simulink model "dspwwv_receiver"  (Simulink 8.3)
settings: Solver=FixedStepDiscrete  StartTime=0.0  StopTime=0  RelTol=1e-3
model workspace (MATLAB code in the model file):
  | MISS = boolean(zeros(1,100)');
  | ZERO =  boolean([ones(1,17) zeros(1,83)]');
  | ONE =  boolean([ones(1,47) zeros(1,53)]');
  | MARKER =  boolean([ones(1,77) zeros(1,23)]');
undefined symbols (not defined in the file or in its folder): magnitude
libraries: dspsigops x9, dspstat3 x2, dspmlti4 x2, dspbuff3 x2, simulink x2, dspsrcs4 x1, dspswit3 x1
settings Model: Creator=The MathWorks Inc.
settings SolverCC: InsertRTBMode=Auto
settings DataIOCC: SaveFormat=Structure
settings OptimizationCC: InlineParams=on  ExpressionDepthLimit=2147483647  InitFltsAndDblsToZero=on  EfficientMapNaN2IntZero=off
settings DebuggingCC: FcnCallInpInsideContextMsg=UseLocalSettings  StrictBusMsg=Warning
settings HardwareCC: ProdIntDivRoundTo=Zero  ProdHWDeviceType=Generic->Unspecified (assume 32-bit Generic)  TargetHWDeviceType=32-bit Generic
settings ModelReferenceCC: ModelReferenceNumInstancesAllowed=Single
settings SFSimCC: SFSimEcho=off  SimParseCustomCode=off

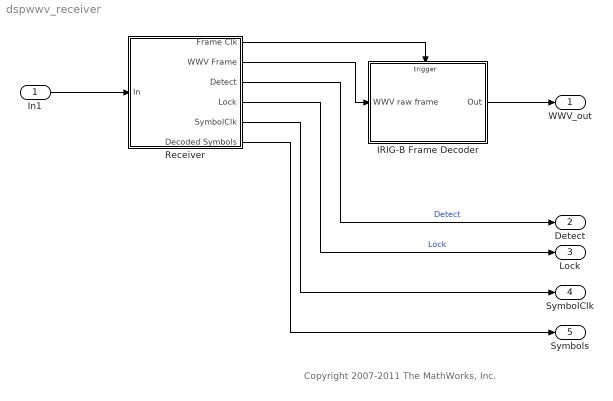
== system dspwwv_receiver ==
  note: Copyright 2007-2011 The MathWorks, Inc.
  In1 : Inport  OutDataTypeStr=single  PortDimensions=[80 1]
  IRIG-B Frame Decoder : Subsystem  TreatAsAtomicUnit=on
      settings: RTWSystemCode=Nonreusable function
  Receiver : Subsystem  TreatAsAtomicUnit=on
      settings: RTWSystemCode=Inline
  WWV_out : Outport
  Detect : Outport  Port=2
  Lock : Outport  Port=3
  SymbolClk : Outport  Port=4
  Symbols : Outport  Port=5
  wires:
  Receiver/4(Lock) -> Lock/1  "Lock"
  Receiver/3(Detect) -> Detect/1  "Detect"
  Receiver/2(WWV Frame) -> IRIG-B Frame Decoder/1(WWV raw frame)
  IRIG-B Frame Decoder/1(Out) -> WWV_out/1
  In1/1 -> Receiver/1(In)
  Receiver/5(SymbolClk) -> SymbolClk/1
  Receiver/6(Decoded Symbols) -> Symbols/1
  Receiver/1(Frame Clk) -> IRIG-B Frame Decoder/Trigger

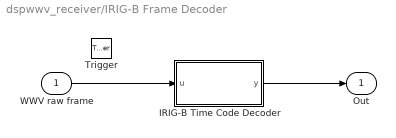
== system dspwwv_receiver/IRIG-B Frame Decoder ==
  WWV raw frame : Inport
  Trigger : TriggerPort  StatesWhenEnabling=reset
  IRIG-B Time Code Decoder : MATLAB Function  TreatAsAtomicUnit=on
  Out : Outport
  wires:
  WWV raw frame/1 -> IRIG-B Time Code Decoder/1(u)
  IRIG-B Time Code Decoder/1(y) -> Out/1

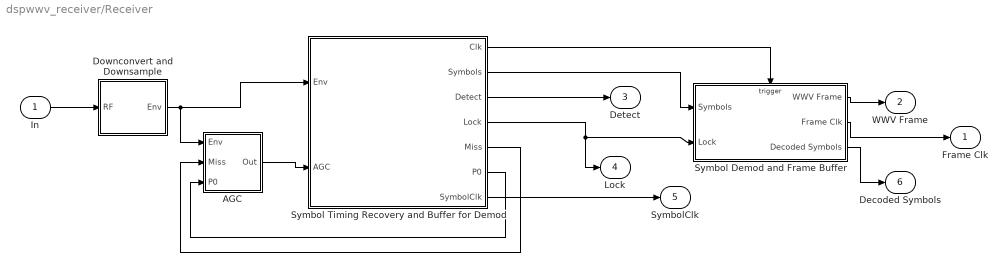
== system dspwwv_receiver/Receiver ==
  In : Inport
  AGC : Subsystem  TreatAsAtomicUnit=on
      settings: MinAlgLoopOccurrences=on  RTWSystemCode=Nonreusable function
  Downconvert and Downsample : Subsystem  TreatAsAtomicUnit=on
      settings: RTWSystemCode=Nonreusable function
  Symbol Demod and Frame Buffer : Subsystem  TreatAsAtomicUnit=on
      settings: RTWSystemCode=Nonreusable function
  Symbol Timing Recovery and Buffer for Demod : Subsystem  TreatAsAtomicUnit=on
      settings: RTWSystemCode=Nonreusable function
  Frame Clk : Outport
  WWV Frame : Outport  Port=2
  Detect : Outport  Port=3
  Lock : Outport  Port=4
  SymbolClk : Outport  Port=5
  Decoded Symbols : Outport  Port=6
  wires:
  Symbol Timing Recovery and Buffer for Demod/1(Clk) -> Symbol Demod and Frame Buffer/Trigger
  Symbol Demod and Frame Buffer/2(Frame Clk) -> Frame Clk/1
  Symbol Demod and Frame Buffer/1(WWV Frame) -> WWV Frame/1
  Symbol Timing Recovery and Buffer for Demod/2(Symbols) -> Symbol Demod and Frame Buffer/1(Symbols)
  Symbol Timing Recovery and Buffer for Demod/6(P0) -> AGC/3(P0)
  Symbol Timing Recovery and Buffer for Demod/5(Miss) -> AGC/2(Miss)
  Symbol Timing Recovery and Buffer for Demod/3(Detect) -> Detect/1
  AGC/1(Out) -> Symbol Timing Recovery and Buffer for Demod/2(AGC)
  In/1 -> Downconvert and Downsample/1(RF)
  Downconvert and Downsample/1(Env) -> Symbol Timing Recovery and Buffer for Demod/1(Env), AGC/1(Env)
  Symbol Timing Recovery and Buffer for Demod/7(SymbolClk) -> SymbolClk/1
  Symbol Timing Recovery and Buffer for Demod/4(Lock) -> Symbol Demod and Frame Buffer/2(Lock), Lock/1
  Symbol Demod and Frame Buffer/3(Decoded Symbols) -> Decoded Symbols/1

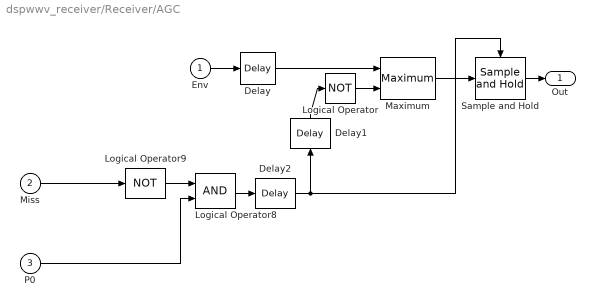
== system dspwwv_receiver/Receiver/AGC ==
  Env : Inport
  Miss : Inport  Port=2
  P0 : Inport  Port=3
  Delay : dspsigops/Delay  dly_unit=Samples  delay=3  ic_detail=off  dif_ic_for_ch=off  dif_ic_for_dly=off  ic=0  reset_popup=None
  Delay1 : dspsigops/Delay  dly_unit=Samples  delay=1  ic_detail=off  dif_ic_for_ch=off  dif_ic_for_dly=off  ic=0  reset_popup=None
  Delay2 : dspsigops/Delay  dly_unit=Samples  delay=1  ic_detail=off  dif_ic_for_ch=off  dif_ic_for_dly=off  ic=0  reset_popup=None
  Logical Operator : Logic  Operator=NOT  Inputs=1
  Logical Operator8 : Logic
  Logical Operator9 : Logic  Operator=NOT  Inputs=1
  Maximum : dspstat3/Maximum  fcn=Running  reset=Non-zero sample  indexBase=One  operateOver=Each column  Dimension=1  colComp=on  operation=maximum  roiEnable=off  roiType=Rectangles  roiPortion=Entire ROI  roiOutput=Individual statistics for each ROI  roiFlag=off  accumDataTypeStr=Inherit: Same as product output  accumLastDataTypeStr=Inherit: Same as product output  roundingMode=Floor  overflowMode=off
  Sample and Hold : dspsigops/Sample and Hold  trig=Falling edge  initCond=single(0.075)  latchinput=off
  Out : Outport
  wires:
  P0/1 -> Logical Operator8/2
  Miss/1 -> Logical Operator9/1
  Sample and Hold/1 -> Out/1
  Env/1 -> Delay/1
  Delay/1 -> Maximum/1
  Delay1/1 -> Logical Operator/1
  Logical Operator/1 -> Maximum/2
  Maximum/1 -> Sample and Hold/1
  Delay2/1 -> Delay1/1, Sample and Hold/Trigger
  Logical Operator8/1 -> Delay2/1
  Logical Operator9/1 -> Logical Operator8/1

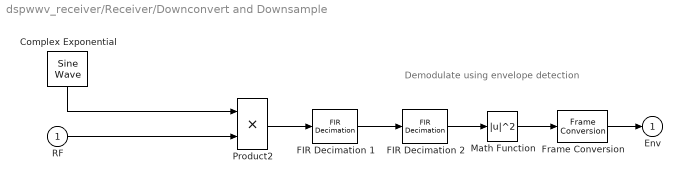
== system dspwwv_receiver/Receiver/Downconvert and Downsample ==
  note: Demodulate using envelope detection
  RF : Inport
  Complex Exponential : dspsrcs4/Sine Wave  Amplitude=1  Frequency=100  Phase=0  SampleMode=Discrete  OutComplex=Complex  CompMethod=Table lookup  TableSize=Memory  SampleTime=1/8000  SamplesPerFrame=80  ResetState=Restart at time zero  dataType=single  wordLen=16  udDataType=sfix(16)  fracBitsMode=Best precision  numFracBits=14  OutDataTypeStr=single  LastOutDataTypeStr=single
      settings: additionalParams=on
  FIR Decimation 1 : dspmlti4/FIR Decimation  h=single(fir1(31, 1/40))  D=20  filtStruct=Direct form  framing=Maintain input frame rate  inputOffset=0  outputBufInitCond=0  InputProcessing=Columns as channels (frame based)  firstCoeffDataTypeStr=Inherit: Same word length as input  firstCoeffLastDataTypeStr=Inherit: Same word length as input  firstCoeffMin=[]  firstCoeffMax=[]  outputDataTypeStr=Inherit: Same as accumulator  outputLastDataTypeStr=Inherit: Same as accumulator  outputMin=[]  outputMax=[]  roundingMode=Floor  overflowMode=off  FilterSource=Specify via dialog  FilterObject=Hm_firdecim
  FIR Decimation 2 : dspmlti4/FIR Decimation  h=single(fir1(15, 1/8))  D=4  filtStruct=Direct form  framing=Maintain input frame rate  inputOffset=0  outputBufInitCond=0  InputProcessing=Columns as channels (frame based)  firstCoeffDataTypeStr=Inherit: Same word length as input  firstCoeffLastDataTypeStr=Inherit: Same word length as input  firstCoeffMin=[]  firstCoeffMax=[]  outputDataTypeStr=Inherit: Same as accumulator  outputLastDataTypeStr=Inherit: Same as accumulator  outputMin=[]  outputMax=[]  roundingMode=Floor  overflowMode=off  FilterSource=Specify via dialog  FilterObject=Hm_firdecim
  Frame Conversion : FrameConversion  OutFrame=Sample-based
  Math Function : Math  Operator=magnitude^2  SaturateOnIntegerOverflow=on
  Product2 : Product  SaturateOnIntegerOverflow=on  InputSameDT=on  OutDataTypeStr=Inherit: Same as first input
  Env : Outport
  wires:
  Frame Conversion/1 -> Env/1
  Math Function/1 -> Frame Conversion/1
  FIR Decimation 2/1 -> Math Function/1
  FIR Decimation 1/1 -> FIR Decimation 2/1
  Product2/1 -> FIR Decimation 1/1
  RF/1 -> Product2/2
  Complex Exponential/1 -> Product2/1

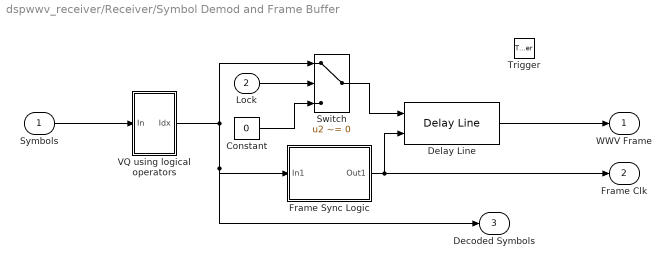
== system dspwwv_receiver/Receiver/Symbol Demod and Frame Buffer ==
  Symbols : Inport
  Lock : Inport  Port=2
  Trigger : TriggerPort  StatesWhenEnabling=reset
  Constant : Constant  Value=0  OutDataTypeStr=int8
  Delay Line : dspbuff3/Delay Line  siz=58  ic=0  directfeed=off  enable_output=on  hold_output=off  TreatMby1Signals=One channel
  Frame Sync Logic : Subsystem
  Switch : Switch  Criteria=u2 ~= 0
  VQ using logical operators : Subsystem
  WWV Frame : Outport
  Frame Clk : Outport  Port=2
  Decoded Symbols : Outport  Port=3
  wires:
  Switch/1 -> Delay Line/1
  Constant/1 -> Switch/3
  Lock/1 -> Switch/2
  Frame Sync Logic/1(Out1) -> Frame Clk/1, Delay Line/2
  Delay Line/1 -> WWV Frame/1
  Symbols/1 -> VQ using logical operators/1(In)
  VQ using logical operators/1(Idx) -> Switch/1, Frame Sync Logic/1(In1), Decoded Symbols/1

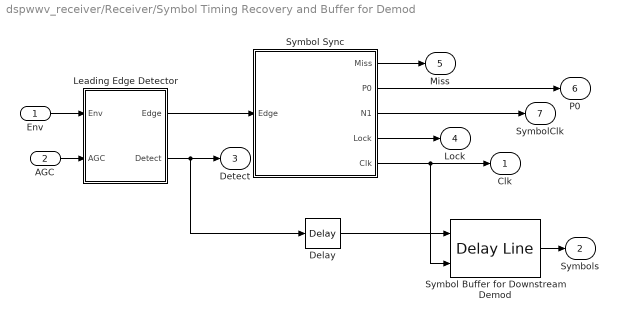
== system dspwwv_receiver/Receiver/Symbol Timing Recovery and Buffer for Demod ==
  Env : Inport
  AGC : Inport  Port=2
  Delay : dspsigops/Delay  dly_unit=Samples  delay=2  ic_detail=off  dif_ic_for_ch=off  dif_ic_for_dly=off  ic=0  reset_popup=None
  Leading Edge Detector : Subsystem
  Symbol Buffer for Downstream Demod : dspbuff3/Delay Line  siz=100  ic=0  directfeed=off  enable_output=on  hold_output=off  TreatMby1Signals=One channel
  Symbol Sync : Stateflow chart  TreatAsAtomicUnit=on
  Clk : Outport
  Symbols : Outport  Port=2
  Detect : Outport  Port=3
  Lock : Outport  Port=4
  Miss : Outport  Port=5
  P0 : Outport  Port=6
  SymbolClk : Outport  Port=7
  wires:
  Symbol Buffer for Downstream Demod/1 -> Symbols/1
  Delay/1 -> Symbol Buffer for Downstream Demod/1
  AGC/1 -> Leading Edge Detector/2(AGC)
  Env/1 -> Leading Edge Detector/1(Env)
  Leading Edge Detector/2(Detect) -> Delay/1, Detect/1
  Symbol Sync/5(" Clk") -> Symbol Buffer for Downstream Demod/2, Clk/1
  Leading Edge Detector/1(Edge) -> Symbol Sync/1(Edge)
  Symbol Sync/1(Miss) -> Miss/1
  Symbol Sync/2(P0) -> P0/1
  Symbol Sync/4(" Lock") -> Lock/1
  Symbol Sync/3(N1) -> SymbolClk/1

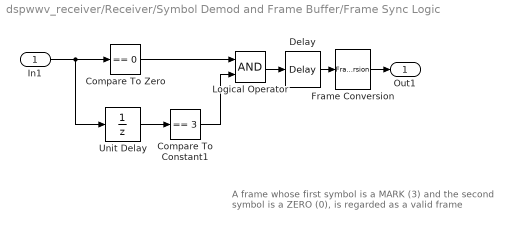
== system dspwwv_receiver/Receiver/Symbol Demod and Frame Buffer/Frame Sync Logic ==
  note: A frame whose first symbol is a MARK (3) and the
      | second symbol is a ZERO (0), is regarded as a valid frame
  In1 : Inport
  Compare To Constant1 : simulink/Logic and Bit Operations/Compare To Constant  relop===  const=3  OutDataTypeStr=uint8  ZeroCross=off
  Compare To Zero : simulink/Logic and Bit Operations/Compare To Zero  relop===  OutDataTypeStr=uint8  ZeroCross=off
  Delay : dspsigops/Delay  dly_unit=Samples  delay=59  ic_detail=off  dif_ic_for_ch=off  dif_ic_for_dly=off  ic=0  reset_popup=None
  Frame Conversion : FrameConversion  OutFrame=Sample-based
  Logical Operator : Logic  AllPortsSameDT=off  OutDataTypeStr=boolean
  Unit Delay : UnitDelay  SampleTime=-1
  Out1 : Outport
  wires:
  Frame Conversion/1 -> Out1/1
  Delay/1 -> Frame Conversion/1
  Compare To Zero/1 -> Logical Operator/1
  In1/1 -> Compare To Zero/1, Unit Delay/1
  Logical Operator/1 -> Delay/1
  Compare To Constant1/1 -> Logical Operator/2
  Unit Delay/1 -> Compare To Constant1/1

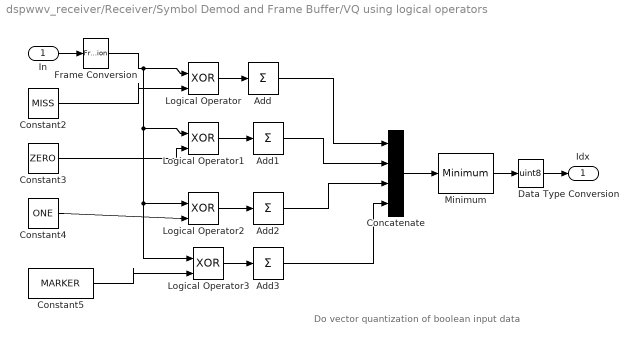
== system dspwwv_receiver/Receiver/Symbol Demod and Frame Buffer/VQ using logical operators ==
  note: Do vector quantization of boolean input data
  In : Inport
  Add{,1..3} (4 alike) : Sum  Inputs=+
  Concatenate : Concatenate  NumInputs=4  ConcatenateDimension=2
  Constant2 : Constant  Value=MISS  VectorParams1D=off  OutDataTypeStr=boolean
  Constant3 : Constant  Value=ZERO  VectorParams1D=off  OutDataTypeStr=boolean
  Constant4 : Constant  Value=ONE  VectorParams1D=off  OutDataTypeStr=boolean
  Constant5 : Constant  Value=MARKER  VectorParams1D=off  OutDataTypeStr=boolean
  Data Type Conversion : DataTypeConversion  OutDataTypeStr=uint8
  Frame Conversion : FrameConversion  OutFrame=Sample-based
  Logical Operator{,1..3} (4 alike) : Logic  Operator=XOR  IconShape=distinctive  AllPortsSameDT=off  OutDataTypeStr=boolean
  Minimum : dspstat3/Minimum  fcn=Index  reset=None  InputProcessing=Columns as channels (frame based)  indexBase=Zero  operateOver=Each column  Dimension=1  colComp=on  operation=minimum  roiEnable=off  roiType=Rectangles  roiPortion=Entire ROI  roiOutput=Individual statistics for each ROI  roiFlag=off  roundingMode=Floor  overflowMode=off
  Idx : Outport
  wires:
  In/1 -> Frame Conversion/1
  Frame Conversion/1 -> Logical Operator3/1, Logical Operator2/1, Logical Operator1/1, Logical Operator/1
  Concatenate/1 -> Minimum/1
  Add3/1 -> Concatenate/4
  Add1/1 -> Concatenate/2
  Logical Operator3/1 -> Add3/1
  Logical Operator2/1 -> Add2/1
  Logical Operator1/1 -> Add1/1
  Constant5/1 -> Logical Operator3/2
  Constant4/1 -> Logical Operator2/2
  Constant3/1 -> Logical Operator1/2
  Add/1 -> Concatenate/1
  Logical Operator/1 -> Add/1
  Constant2/1 -> Logical Operator/2
  Minimum/1 -> Data Type Conversion/1
  Data Type Conversion/1 -> Idx/1
  Add2/1 -> Concatenate/3

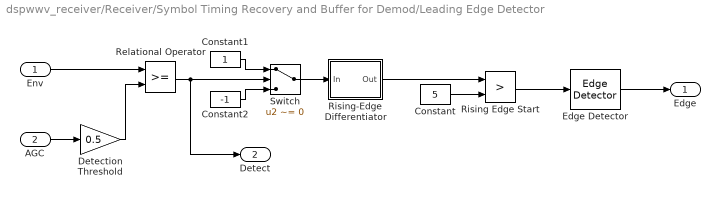
== system dspwwv_receiver/Receiver/Symbol Timing Recovery and Buffer for Demod/Leading Edge Detector ==
  Env : Inport
  AGC : Inport  Port=2
  Constant : Constant  Value=5  OutDataTypeStr=int8
  Constant1 : Constant  OutDataTypeStr=int8
  Constant2 : Constant  Value=-1  OutDataTypeStr=int8
  Detection Threshold : Gain  Gain=0.5  SaturateOnIntegerOverflow=on  OutDataTypeStr=Inherit: Same as input  ParamDataTypeStr=Inherit: Same as input
  Edge Detector : dspswit3/Edge Detector
  Relational Operator : RelationalOperator  InputSameDT=on
  Rising Edge Start : RelationalOperator  Operator=>  OutDataTypeStr=boolean  ZeroCross=off
  Rising-Edge Differentiator : Subsystem
  Switch : Switch  Criteria=u2 ~= 0  ZeroCross=off
  Edge : Outport
  Detect : Outport  Port=2
  wires:
  Constant2/1 -> Switch/3
  Constant1/1 -> Switch/1
  Rising-Edge Differentiator/1(Out) -> Rising Edge Start/1
  Switch/1 -> Rising-Edge Differentiator/1(In)
  Constant/1 -> Rising Edge Start/2
  Env/1 -> Relational Operator/1
  Rising Edge Start/1 -> Edge Detector/1
  Edge Detector/1 -> Edge/1
  Relational Operator/1 -> Switch/2, Detect/1
  Detection Threshold/1 -> Relational Operator/2
  AGC/1 -> Detection Threshold/1

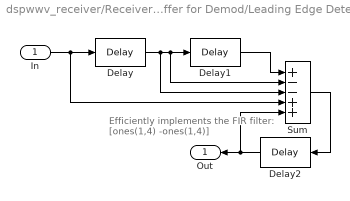
== system dspwwv_receiver/Receiver/Symbol Timing Recovery and Buffer for Demod/Leading Edge Detector/Rising-Edge Differentiator ==
  note: Efficiently implements the FIR filter:
      | [ones(1,4) -ones(1,4)]
  In : Inport
  Delay : dspsigops/Delay  dly_unit=Samples  delay=4  ic_detail=off  dif_ic_for_ch=off  dif_ic_for_dly=off  ic=0  reset_popup=None
  Delay1 : dspsigops/Delay  dly_unit=Samples  delay=4  ic_detail=off  dif_ic_for_ch=off  dif_ic_for_dly=off  ic=0  reset_popup=None
  Delay2 : dspsigops/Delay  dly_unit=Samples  delay=1  ic_detail=off  dif_ic_for_ch=off  dif_ic_for_dly=off  ic=0  reset_popup=None
  Sum : Sum  Inputs=+--++
  Out : Outport
  wires:
  Delay1/1 -> Sum/1
  Delay2/1 -> Out/1, Sum/5
  Sum/1 -> Delay2/1
  Delay/1 -> Sum/3, Sum/2, Delay1/1
  In/1 -> Delay/1, Sum/4

== stateflow chart Receiver/Symbol Timing Recovery and Buffer for Demod/Symbol Sync ==
  settings: sampleTime=0.01
  state Integration [parallel]
    settings: executionOrder=2
    state Running
      Running -> (junction 18) [order 1] : at(NZero,tick)
          | {P0=0}
    state Disabled
    Disabled -> Running : tick
    Running -> Disabled [order 1] : en(SymbolSync.Lock.Sync)
        | {P0=1}
    (default) -> Disabled
  state Clock [parallel]
    settings: executionOrder=3
    state ClkLo
    state Clk
    state Rst
    Clock -> Rst : en(SymbolSync.Lock.Sync)
    (default) -> Rst
    Rst -> Clk
    Clk -> ClkLo
    ClkLo -> Clk : every(N1,tick)
        | [ in(SymbolSync.Search) ]
  state SymbolSync [parallel]
    settings: executionOrder=1
    state Search
      state SeekSilence
      state Wait
      state FindPulse
        en: cnt=Nwin
        du: cnt--
      SeekSilence -> SeekSilence [order 2] : [Edge]
      Wait -> SeekSilence : [Edge]
      SeekSilence -> SymbolSync.Search.FindPulse [order 1] : after(N1est-Nhalfwin+1,tick)
      SymbolSync.Search.FindPulse -> Wait [order 2] : [cnt==0]
    state Lock
      state Sync
      state FindPulse
        en: cnt=Nwin
        du: cnt--
      SymbolSync.Lock.FindPulse -> (junction 41) [order 2] : [cnt==0]
      SymbolSync.Lock.FindPulse -> (junction 42) [order 1] : [Edge]
      (junction 41) -> Sync [order 2] : {Miss=1
          | dly=N1-Nwin-2}
      (junction 42) -> Sync : {Miss = 0
          | N1 += Nhalfwin-cnt
          | dly=N1-Nhalfwin+1}
      Sync -> SymbolSync.Lock.FindPulse : after(dly,tick)
    (default) -> Wait
    (junction 41) -> Wait [order 1] : [Miss]
    SymbolSync.Search.FindPulse -> (junction 42) [order 1] : [Edge]
        | {N1=N1est}
  data: NZero constant int16 =17; cnt local int16 [0..127]; N1est constant int16 =100; Nwin constant int16 =11; Nhalfwin local int16 [0..5] =6; dly local int16; Edge input boolean [0..1]; Miss output boolean [0..1]; P0 output boolean [0..1]; N1 output int16 [0..1023] =100; Lock output boolean; Clk output boolean
  data NZero settings: description=Number of samples in ZERO bit (AGC) integration window
  data N1est settings: description=Estimated of number of samples per bit interval (1 second, i.e., 50 for 50Hz nominal sample frequency)
  data Nwin settings: description=Track window, in samples
  data Nhalfwin settings: description=Half of Nwin, (Nwin+1)/2
  data N1 settings: description=Number of samples per bit interval (1 second), corrected during track

== matlab function IRIG-B Frame Decoder/IRIG-B Time Code Decoder ==
  data: u input uint8 size=[58 1]; y output single size=[7 1]
function y  = IRIG_B(u)
% Interpret IRIG-B data frame and convert to time code.
%
% Input u: 58x1 int8
%   It has already been detected that this is a valid frame that
%   needs to be decoded, based on the first and second symbol values which 
%   are 3 and 0 respectively. We only decode the remaining 58 symbol 
%   values of the 60 symbol frame. 
%   Each element of input u is one of four IRIG code values,
%   where the values 0-3 correspond to the symbols
%   0:MISS   (no 100Hz audio pulse found)
%   1:ZERO   (0.1 sec pulse)
%   2:ONE    (0.3 sec pulse)
%   3:MARKER (0.7 sec pulse)
%
% Output y: 7x1 double
%   Each element of output y is an element of the time code,
%   1:UTC time (24-hour time, MM.SS)
%   2:UT1 time correction
%   3:Year (>=2000)
%   4:Day of year
%   5:Daylight savings indicator #1
%   6:Daylight savings indicator #2
%   7:Leap second indicator

y = single(zeros(7,1));  % Initialize output vector
y(6)  = single(isONE(u(2)));
y(7)  = single(isONE(u(3)));
yy    = get_bcd(u,4,4);
mm    = get_bcd(u,10,7);
hh    = get_bcd(u,20,6);
y(1)  = single(100*hh + mm);
y(4)  = single(get_bcd(u,30,10));
utneg = isONE(u(50));
y(3)  = single(2000 + yy + 10*get_bcd(u,51,4));
y(5)  = single(isONE(u(55)));
if utneg, utfac=-0.1; else utfac=0.1; end
y(2)  = single(utfac*double(get_bcd(u,56,3)));

% --------------------------------
function s = get_bcd(x,j,N)
% Convert input X to BCD using N bits
% Start converting from x(j)

bcd = int16([1,2,4,8,10,20,40,80,100,200]);
s = int16(0); % BCD accumulator
if N>int16(10), N=int16(10); end % Protect from too many bits
Nx = int16(numel(x));
for i=1:N
    if j>Nx, break; end
    % Count current input element as "on"
    % if it is either P_ONE or P_ID
    if isONE(x(j))
        s = s + bcd(i);
    end
    j=j+1;  % next input bit
    if (i==4)||(i==8)
        j=j+1;  % also skip next unused P0 bit
    end
end

% ---------------------------
function y = isONE(x)
% TRUE if input symbol is P_ONE or P_ID
y = (x==2) || (x==3);

% [EOF]
